simulink library "CTRL_SPECCTRL_FB_FUS"  (R2024b)
settings: Solver=VariableStepAuto  StartTime=0.0  StopTime=10.0  RelTol=1e-3
settings Model: Creator=blatak  LastModifiedBy=blatak

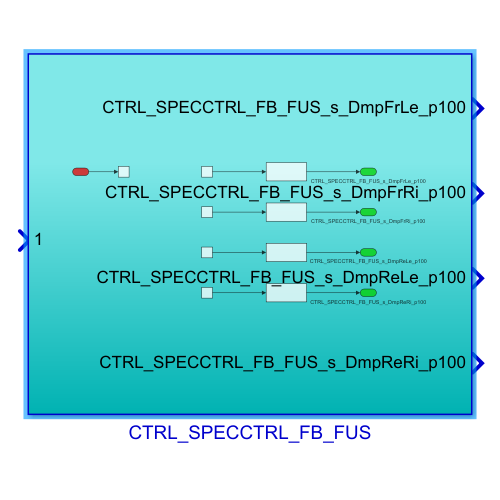
[thumbnail: Simulink's stored preview of the top-level diagram]
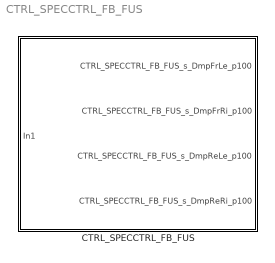
== system CTRL_SPECCTRL_FB_FUS ==
  CTRL_SPECCTRL_FB_FUS : Subsystem

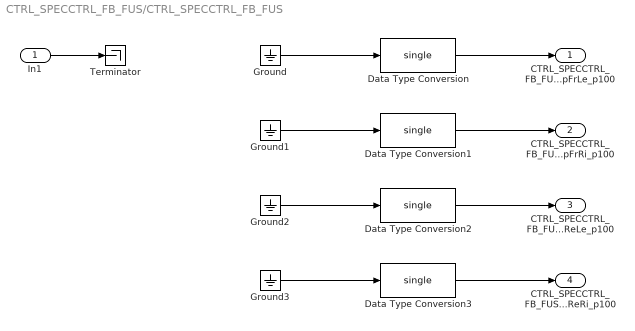
== system CTRL_SPECCTRL_FB_FUS/CTRL_SPECCTRL_FB_FUS ==
  In1 : Inport
  Data Type Conversion{,1..3} (4 alike) : DataTypeConversion  OutDataTypeStr=single  SaturateOnIntegerOverflow=off  RndMeth=Floor
  Ground{,1..3} (4 alike) : Ground
  Terminator : Terminator
  CTRL_SPECCTRL_FB_FUS_s_DmpFrLe_p100 : Outport
  CTRL_SPECCTRL_FB_FUS_s_DmpFrRi_p100 : Outport  Port=2
  CTRL_SPECCTRL_FB_FUS_s_DmpReLe_p100 : Outport  Port=3
  CTRL_SPECCTRL_FB_FUS_s_DmpReRi_p100 : Outport  Port=4
  wires:
  Ground/1 -> Data Type Conversion/1
  Data Type Conversion/1 -> CTRL_SPECCTRL_FB_FUS_s_DmpFrLe_p100/1
  Ground1/1 -> Data Type Conversion1/1
  Ground2/1 -> Data Type Conversion2/1
  Ground3/1 -> Data Type Conversion3/1
  Data Type Conversion1/1 -> CTRL_SPECCTRL_FB_FUS_s_DmpFrRi_p100/1
  Data Type Conversion2/1 -> CTRL_SPECCTRL_FB_FUS_s_DmpReLe_p100/1
  Data Type Conversion3/1 -> CTRL_SPECCTRL_FB_FUS_s_DmpReRi_p100/1
  In1/1 -> Terminator/1
